simulink model "FirstPass"  (R2017b)
settings: Solver=FixedStepAuto  StartTime=0.0  StopTime=10.0  FixedStep=0.08  RelTol=1e-3
model workspace (MAT data in the model file):
  ContractValidatorBlocksMap = containers.Map
  ContractValidatorBlocksMap.serialization.keys = {'FirstPass/Req_s3_1_2_2_p19_2/validator', 'FirstPass/Req_s3_1_2_2_p19_3/validator', 'FirstPass/contract/validator', 'FirstPass/contract1/validator'}
  ContractValidatorBlocksMap.serialization.values{1}.block = 'FirstPass/Req_s3_1_2_2_p19_2/validator'
  ContractValidatorBlocksMap.serialization.values{1}.assumePorts = 0
  ContractValidatorBlocksMap.serialization.values{1}.guaranteePorts = 1
  ContractValidatorBlocksMap.serialization.values{1}.modeBlocksPorts = 0
  ContractValidatorBlocksMap.serialization.values{1}.portHandles.Inport = 2748.11108398
  ContractValidatorBlocksMap.serialization.values{1}.portHandles.Outport = 2749.11108398
  ContractValidatorBlocksMap.serialization.values{1}.portHandles.Enable = []
  ContractValidatorBlocksMap.serialization.values{1}.portHandles.Trigger = []
  ContractValidatorBlocksMap.serialization.values{1}.portHandles.State = []
  ContractValidatorBlocksMap.serialization.values{1}.portHandles.LConn = []
  ContractValidatorBlocksMap.serialization.values{1}.portHandles.RConn = []
  ContractValidatorBlocksMap.serialization.values{1}.portHandles.Ifaction = []
  ContractValidatorBlocksMap.serialization.values{1}.portHandles.Reset = []
  ContractValidatorBlocksMap.serialization.values{1}.portConnectivity(1).Type = '1'
  ContractValidatorBlocksMap.serialization.values{1}.portConnectivity(1).Position = [365 90]
  ContractValidatorBlocksMap.serialization.values{1}.portConnectivity(1).SrcBlock = 2685.11108398
  ContractValidatorBlocksMap.serialization.values{1}.portConnectivity(1).SrcPort = 0
  ContractValidatorBlocksMap.serialization.values{1}.portConnectivity(1).DstBlock = []
  ContractValidatorBlocksMap.serialization.values{1}.portConnectivity(1).DstPort = []
  ContractValidatorBlocksMap.serialization.values{1}.portConnectivity(2).Type = '1'
  ContractValidatorBlocksMap.serialization.values{1}.portConnectivity(2).Position = [500 90]
  ContractValidatorBlocksMap.serialization.values{1}.portConnectivity(2).SrcBlock = []
  ContractValidatorBlocksMap.serialization.values{1}.portConnectivity(2).SrcPort = []
  ContractValidatorBlocksMap.serialization.values{1}.portConnectivity(2).DstBlock = 2694.11108398
  ContractValidatorBlocksMap.serialization.values{1}.portConnectivity(2).DstPort = 0
  ContractValidatorBlocksMap.serialization.values{2}.block = 'FirstPass/Req_s3_1_2_2_p19_3/validator'
  ContractValidatorBlocksMap.serialization.values{2}.assumePorts = 0
  ContractValidatorBlocksMap.serialization.values{2}.guaranteePorts = 1
  ContractValidatorBlocksMap.serialization.values{2}.modeBlocksPorts = 0
  ContractValidatorBlocksMap.serialization.values{2}.portHandles.Inport = 2746.11132812
  ContractValidatorBlocksMap.serialization.values{2}.portHandles.Outport = 2747.11108398
  ContractValidatorBlocksMap.serialization.values{2}.portHandles.Enable = []
  ContractValidatorBlocksMap.serialization.values{2}.portHandles.Trigger = []
  ContractValidatorBlocksMap.serialization.values{2}.portHandles.State = []
  ContractValidatorBlocksMap.serialization.values{2}.portHandles.LConn = []
  ContractValidatorBlocksMap.serialization.values{2}.portHandles.RConn = []
  ContractValidatorBlocksMap.serialization.values{2}.portHandles.Ifaction = []
  ContractValidatorBlocksMap.serialization.values{2}.portHandles.Reset = []
  ContractValidatorBlocksMap.serialization.values{2}.portConnectivity(1).Type = '1'
  ContractValidatorBlocksMap.serialization.values{2}.portConnectivity(1).Position = [365 75]
  ContractValidatorBlocksMap.serialization.values{2}.portConnectivity(1).SrcBlock = 2703.11108398
  ContractValidatorBlocksMap.serialization.values{2}.portConnectivity(1).SrcPort = 0
  ContractValidatorBlocksMap.serialization.values{2}.portConnectivity(1).DstBlock = []
  ContractValidatorBlocksMap.serialization.values{2}.portConnectivity(1).DstPort = []
  ContractValidatorBlocksMap.serialization.values{2}.portConnectivity(2).Type = '1'
  ContractValidatorBlocksMap.serialization.values{2}.portConnectivity(2).Position = [500 75]
  ContractValidatorBlocksMap.serialization.values{2}.portConnectivity(2).SrcBlock = []
  ContractValidatorBlocksMap.serialization.values{2}.portConnectivity(2).SrcPort = []
  ContractValidatorBlocksMap.serialization.values{2}.portConnectivity(2).DstBlock = 2720.11108398
  ContractValidatorBlocksMap.serialization.values{2}.portConnectivity(2).DstPort = 0
  ContractValidatorBlocksMap.serialization.values{3}.block = 'FirstPass/contract/validator'
  ContractValidatorBlocksMap.serialization.values{3}.assumePorts = 0
  ContractValidatorBlocksMap.serialization.values{3}.guaranteePorts = 1
  ContractValidatorBlocksMap.serialization.values{3}.modeBlocksPorts = 0
  ContractValidatorBlocksMap.serialization.values{3}.portHandles.Inport = 1491.35229492
  ContractValidatorBlocksMap.serialization.values{3}.portHandles.Outport = 1492.35205078
  ContractValidatorBlocksMap.serialization.values{3}.portHandles.Enable = []
  ContractValidatorBlocksMap.serialization.values{3}.portHandles.Trigger = []
  ContractValidatorBlocksMap.serialization.values{3}.portHandles.State = []
  ContractValidatorBlocksMap.serialization.values{3}.portHandles.LConn = []
  ContractValidatorBlocksMap.serialization.values{3}.portHandles.RConn = []
  ContractValidatorBlocksMap.serialization.values{3}.portHandles.Ifaction = []
  ContractValidatorBlocksMap.serialization.values{3}.portHandles.Reset = []
  ContractValidatorBlocksMap.serialization.values{3}.portConnectivity(1).Type = '1'
  ContractValidatorBlocksMap.serialization.values{3}.portConnectivity(1).Position = [365 75]
  ContractValidatorBlocksMap.serialization.values{3}.portConnectivity(1).SrcBlock = 1448.35205078
  ContractValidatorBlocksMap.serialization.values{3}.portConnectivity(1).SrcPort = 0
  ContractValidatorBlocksMap.serialization.values{3}.portConnectivity(1).DstBlock = []
  ContractValidatorBlocksMap.serialization.values{3}.portConnectivity(1).DstPort = []
  ContractValidatorBlocksMap.serialization.values{3}.portConnectivity(2).Type = '1'
  ContractValidatorBlocksMap.serialization.values{3}.portConnectivity(2).Position = [500 75]
  ContractValidatorBlocksMap.serialization.values{3}.portConnectivity(2).SrcBlock = []
  ContractValidatorBlocksMap.serialization.values{3}.portConnectivity(2).SrcPort = []
  ContractValidatorBlocksMap.serialization.values{3}.portConnectivity(2).DstBlock = 1465.35205078
  ContractValidatorBlocksMap.serialization.values{3}.portConnectivity(2).DstPort = 0
  ContractValidatorBlocksMap.serialization.values{4}.block = 'FirstPass/contract1/validator'
  ContractValidatorBlocksMap.serialization.values{4}.assumePorts = 0
  ContractValidatorBlocksMap.serialization.values{4}.guaranteePorts = 1
  ContractValidatorBlocksMap.serialization.values{4}.modeBlocksPorts = 0
  ContractValidatorBlocksMap.serialization.values{4}.portHandles.Inport = 5485.11975098
  ContractValidatorBlocksMap.serialization.values{4}.portHandles.Outport = 5486.11975098
  ContractValidatorBlocksMap.serialization.values{4}.portHandles.Enable = []
  ContractValidatorBlocksMap.serialization.values{4}.portHandles.Trigger = []
  ContractValidatorBlocksMap.serialization.values{4}.portHandles.State = []
  ContractValidatorBlocksMap.serialization.values{4}.portHandles.LConn = []
  ContractValidatorBlocksMap.serialization.values{4}.portHandles.RConn = []
  ContractValidatorBlocksMap.serialization.values{4}.portHandles.Ifaction = []
  ContractValidatorBlocksMap.serialization.values{4}.portHandles.Reset = []
  ContractValidatorBlocksMap.serialization.values{4}.portConnectivity(1).Type = '1'
  ContractValidatorBlocksMap.serialization.values{4}.portConnectivity(1).Position = [365 75]
  ContractValidatorBlocksMap.serialization.values{4}.portConnectivity(1).SrcBlock = 5292.11987305
  ContractValidatorBlocksMap.serialization.values{4}.portConnectivity(1).SrcPort = 0
  ContractValidatorBlocksMap.serialization.values{4}.portConnectivity(1).DstBlock = []
  ContractValidatorBlocksMap.serialization.values{4}.portConnectivity(1).DstPort = []
  ContractValidatorBlocksMap.serialization.values{4}.portConnectivity(2).Type = '1'
  ContractValidatorBlocksMap.serialization.values{4}.portConnectivity(2).Position = [500 75]
  ContractValidatorBlocksMap.serialization.values{4}.portConnectivity(2).SrcBlock = []
  ContractValidatorBlocksMap.serialization.values{4}.portConnectivity(2).SrcPort = []
  ContractValidatorBlocksMap.serialization.values{4}.portConnectivity(2).DstBlock = 5462.12011719
  ContractValidatorBlocksMap.serialization.values{4}.portConnectivity(2).DstPort = 0
  ContractValidatorBlocksMap.serialization.uniformity = 0
  ContractValidatorBlocksMap.serialization.keyType = 'char'
  ContractValidatorBlocksMap.serialization.valueType = 'any'
undefined symbols (not defined in the file or in its folder): contractAfterSimulation, contractBeforeSimulation, ContractBlock, ContractGuaranteeBlock, ContractValidatorBlock, Req_s3_1_2_2_p19_2, saveValidatorParameters
libraries: sldvlib x2
settings Model: Creator=hbourbou  LastModifiedBy=hbourbou

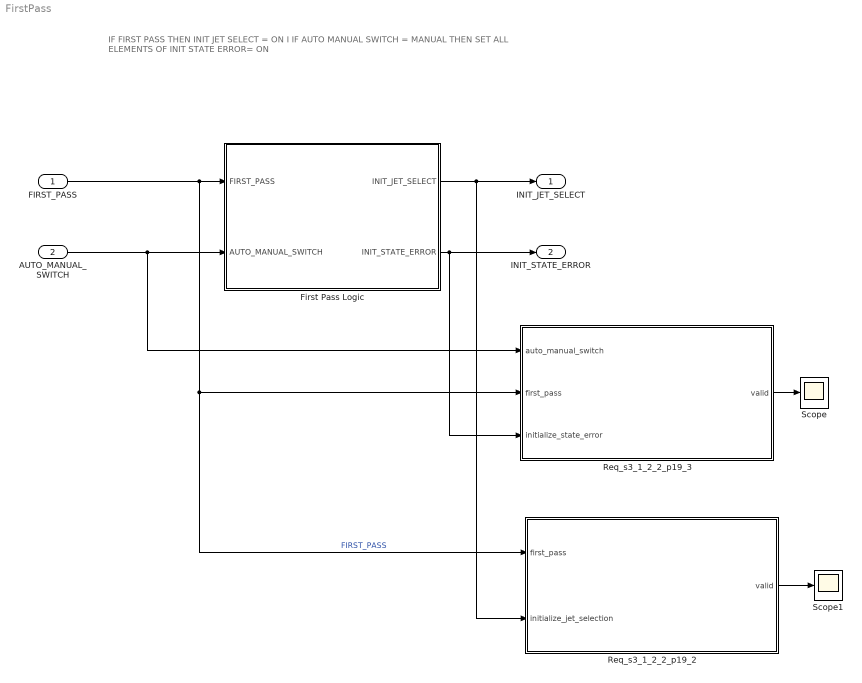
== system FirstPass ==
  note: IF FIRST PASS THEN
      | INIT JET SELECT = ON I
      | IF AUTO MANUAL SWITCH = MANUAL THEN
      | SET ALL ELEMENTS OF INIT STATE ERROR= ON
  FIRST_PASS : Inport  OutDataTypeStr=boolean
  AUTO_MANUAL_SWITCH : Inport  Port=2  OutDataTypeStr=boolean  PortDimensions=1
  First Pass Logic : Subsystem
  Req_s3_1_2_2_p19_2 : Subsystem  mask(ContractBlock){ContractBlockType=Req_s3_1_2_2_p19_2}
      mask init:
      | set_param(gcb, 'LinkStatus', 'none');
      settings: CopyFcn=set_param(gcb, 'LinkStatus', 'none');
      mask DialogControl DescTextVar Prompt: Contract block
      mask Display:
      | text(0.5, 0.5, '{\bf\fontsize{20}Contract}', 'hor', 'center', 'texmode','on');
      | blocks = find_system(gcb, 'LookUnderMasks','all', 'SearchDepth',1,'BlockType','Inport');
      | for i = 1 : length(blocks)
      |     blockName = get_param(blocks(i), 'Name');
      |     [path, blockName] = fileparts(char(blockName));
      |     port_label('input', i, blockName);
      | end
      | 
      | blocks = find_system(gcb, 'LookUnderMasks','all', 'SearchDepth',1,'BlockType','Outport');
      | for i = 1 : length(blocks)
      |     blockName = get_param(blocks(i), 'Name');
      |     [path, blockName] = fileparts(char(blockName));
      |     port_label('output', i, blockName);
      | end
  Req_s3_1_2_2_p19_3 : Subsystem  mask(ContractBlock){ContractBlockType=ContractBlock}
      mask init:
      | set_param(gcb, 'LinkStatus', 'none');
      settings: CopyFcn=set_param(gcb, 'LinkStatus', 'none');
      mask DialogControl DescTextVar Prompt: Contract block
      mask Display:
      | text(0.5, 0.5, '{\bf\fontsize{20}Contract}', 'hor', 'center', 'texmode','on');
      | blocks = find_system(gcb, 'LookUnderMasks','all', 'SearchDepth',1,'BlockType','Inport');
      | for i = 1 : length(blocks)
      |     blockName = get_param(blocks(i), 'Name');
      |     [path, blockName] = fileparts(char(blockName));
      |     port_label('input', i, blockName);
      | end
      | 
      | blocks = find_system(gcb, 'LookUnderMasks','all', 'SearchDepth',1,'BlockType','Outport');
      | for i = 1 : length(blocks)
      |     blockName = get_param(blocks(i), 'Name');
      |     [path, blockName] = fileparts(char(blockName));
      |     port_label('output', i, blockName);
      | end
  Scope : Scope
  Scope1 : Scope
  INIT_JET_SELECT : Outport
  INIT_STATE_ERROR : Outport  Port=2
  wires:
  FIRST_PASS/1 -> Req_s3_1_2_2_p19_2/1(first_pass), Req_s3_1_2_2_p19_3/2(first_pass), First Pass Logic/1(FIRST_PASS)  "FIRST_PASS"
  AUTO_MANUAL_SWITCH/1 -> Req_s3_1_2_2_p19_3/1(auto_manual_switch), First Pass Logic/2(AUTO_MANUAL_SWITCH)
  First Pass Logic/1(INIT_JET_SELECT) -> Req_s3_1_2_2_p19_2/2(initialize_jet_selection), INIT_JET_SELECT/1
  First Pass Logic/2(INIT_STATE_ERROR) -> Req_s3_1_2_2_p19_3/3(initialize_state_error), INIT_STATE_ERROR/1
  Req_s3_1_2_2_p19_3/1(valid) -> Scope/1
  Req_s3_1_2_2_p19_2/1(valid) -> Scope1/1

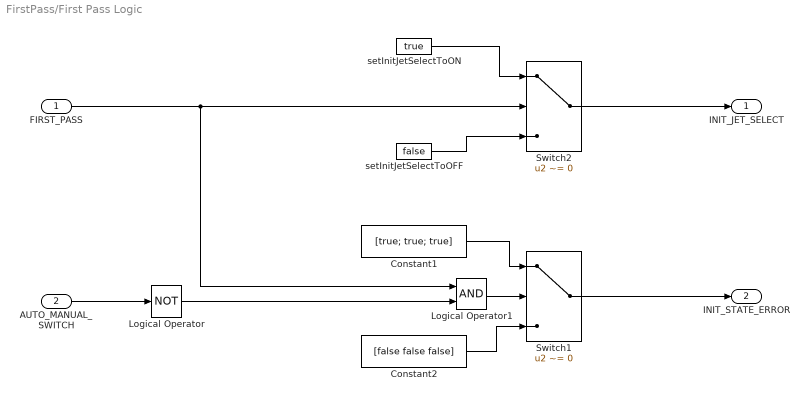
== system FirstPass/First Pass Logic ==
  FIRST_PASS : Inport
  AUTO_MANUAL_SWITCH : Inport  Port=2
  Constant1 : Constant  Value=[true; true; true]  OutDataTypeStr=boolean
  Constant2 : Constant  Value=[false false false]  OutDataTypeStr=boolean
  Logical Operator : Logic  Operator=NOT  AllPortsSameDT=off  OutDataTypeStr=boolean
  Logical Operator1 : Logic  AllPortsSameDT=off  OutDataTypeStr=boolean
  Switch1 : Switch  Criteria=u2 ~= 0
  Switch2 : Switch  Criteria=u2 ~= 0
  setInitJetSelectToOFF : Constant  Value=false  OutDataTypeStr=boolean
  setInitJetSelectToON : Constant  Value=true  OutDataTypeStr=boolean
  INIT_JET_SELECT : Outport
  INIT_STATE_ERROR : Outport  Port=2
  wires:
  Constant1/1 -> Switch1/1
  Switch1/1 -> INIT_STATE_ERROR/1
  Constant2/1 -> Switch1/3
  Switch2/1 -> INIT_JET_SELECT/1
  setInitJetSelectToON/1 -> Switch2/1
  setInitJetSelectToOFF/1 -> Switch2/3
  Logical Operator1/1 -> Switch1/2
  AUTO_MANUAL_SWITCH/1 -> Logical Operator/1
  Logical Operator/1 -> Logical Operator1/2
  FIRST_PASS/1 -> Logical Operator1/1, Switch2/2

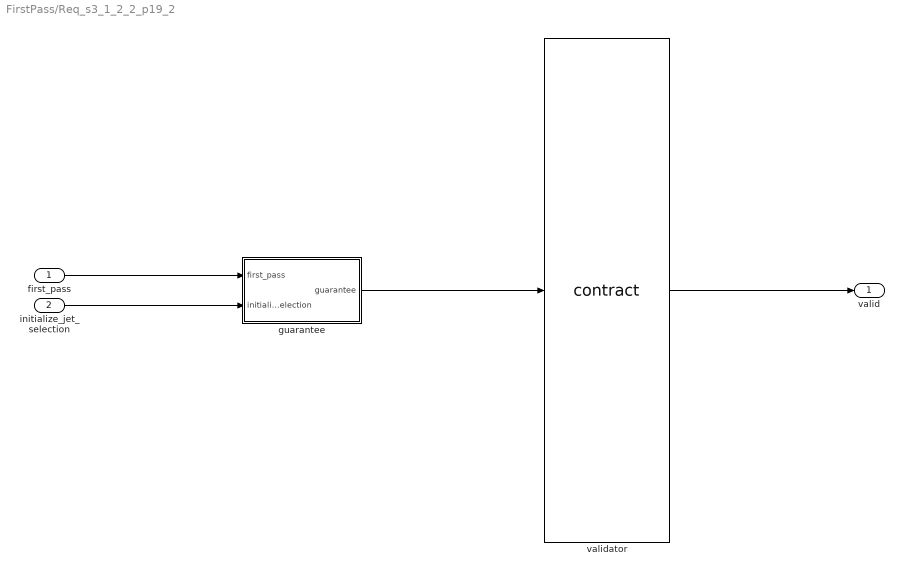
== system FirstPass/Req_s3_1_2_2_p19_2 ==
  first_pass : Inport
  initialize_jet_selection : Inport  Port=2
  guarantee : Subsystem  mask(ContractGuaranteeBlock){ContractBlockType=ContractGuaranteeBlock}
      mask init:
      | set_param(gcb, 'LinkStatus', 'none');
      mask DialogControl DescTextVar Prompt: Guarantee block
  validator : M-S-Function  LoadFcn=saveValidatorParameters(gcb);  InitFcn=contractBeforeSimulation();  StopFcn=contractAfterSimulation();  FunctionName=contract  mask(ContractValidatorBlock){assumePorts=0, guaranteePorts=1, modePorts=0, ContractBlockType=ContractValidatorBlock, createInportsCheckbox=off}
      mask prompts: assumePorts "Assume ports     :"; guaranteePorts "Guarantee ports :"; modePorts "Mode ports        :"; createInportsCheckbox "Create inports and connect them automatically"
      mask init:
      | set_param(gcb,'LinkStatus','none');
      | contract_callback('inputs_callback',gcb);
      mask DialogControl DescTextVar Prompt: The validator block implements the following logic: <br> <br> <b>Sofar</b>(assume<sub>1</sub> <b>&#8743;</b> assume<sub>2</sub> <b>&#8743;</b> ... assume<sub>k</sub>) <b>&rarr;</b> (guarantee<sub>1</sub> <b>&#8743;</b> guarantee<sub>2</sub> <b>&#8743;</b> ... guarantee<sub>m</sub> <b>&#8743;</b>  mode<sub>1</sub> <b>&#8743;</b> mode<sub>2</sub> <b>&#8743;</b> ... <b>&#8743;</b> mode<sub>n</sub> )<br> where mode<sub>i</sub> = require<sub>i</sub> <b>&rarr;</b> ensure<sub>i</sub>
      mask Display:
      | color('black');
      | port_label('input',1,'guarantee');
      | port_label('output',1,'valid');
  valid : Outport
  wires:
  initialize_jet_selection/1 -> guarantee/2(initialize_jet_selection)
  first_pass/1 -> guarantee/1(first_pass)
  validator/1 -> valid/1
  guarantee/1(guarantee) -> validator/1

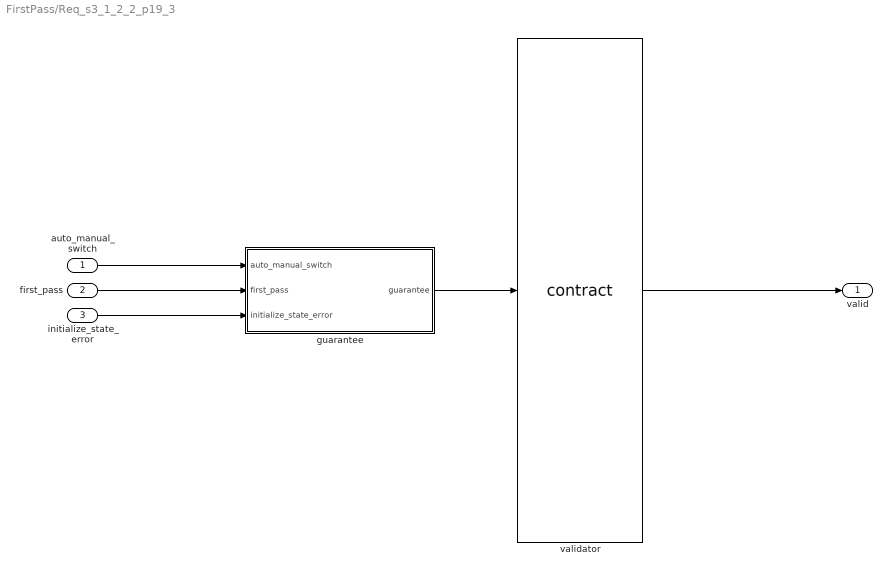
== system FirstPass/Req_s3_1_2_2_p19_3 ==
  auto_manual_switch : Inport
  first_pass : Inport  Port=2
  initialize_state_error : Inport  Port=3
  guarantee : Subsystem  mask(ContractGuaranteeBlock){ContractBlockType=ContractGuaranteeBlock}
      mask init:
      | set_param(gcb, 'LinkStatus', 'none');
      mask DialogControl DescTextVar Prompt: Guarantee block
  validator : M-S-Function  LoadFcn=saveValidatorParameters(gcb);  InitFcn=contractBeforeSimulation();  StopFcn=contractAfterSimulation();  FunctionName=contract  mask(ContractValidatorBlock){assumePorts=0, guaranteePorts=1, modePorts=0, ContractBlockType=ContractValidatorBlock, createInportsCheckbox=on}
      mask prompts: assumePorts "Assume ports     :"; guaranteePorts "Guarantee ports :"; modePorts "Mode ports        :"; createInportsCheckbox "Create inports and connect them automatically"
      mask init:
      | set_param(gcb,'LinkStatus','none');
      | contract_callback('inputs_callback',gcb);
      mask DialogControl DescTextVar Prompt: The validator block implements the following logic: <br> <br> <b>Sofar</b>(assume<sub>1</sub> <b>&#8743;</b> assume<sub>2</sub> <b>&#8743;</b> ... assume<sub>k</sub>) <b>&rarr;</b> (guarantee<sub>1</sub> <b>&#8743;</b> guarantee<sub>2</sub> <b>&#8743;</b> ... guarantee<sub>m</sub> <b>&#8743;</b>  mode<sub>1</sub> <b>&#8743;</b> mode<sub>2</sub> <b>&#8743;</b> ... <b>&#8743;</b> mode<sub>n</sub> )<br> where mode<sub>i</sub> = require<sub>i</sub> <b>&rarr;</b> ensure<sub>i</sub>
      mask Display:
      | color('black');
      | port_label('input',1,'guarantee');
      | port_label('output',1,'valid');
  valid : Outport
  wires:
  first_pass/1 -> guarantee/2(first_pass)
  auto_manual_switch/1 -> guarantee/1(auto_manual_switch)
  validator/1 -> valid/1
  guarantee/1(guarantee) -> validator/1
  initialize_state_error/1 -> guarantee/3(initialize_state_error)

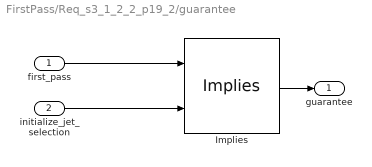
== system FirstPass/Req_s3_1_2_2_p19_2/guarantee ==
  first_pass : Inport
  initialize_jet_selection : Inport  Port=2
  Implies : sldvlib/Verification Utilities/Implies
      settings: SourceProductName=Simulink Design Verifier  SourceProductBaseCode=DV
  guarantee : Outport  OutDataTypeStr=boolean
  wires:
  Implies/1 -> guarantee/1
  first_pass/1 -> Implies/1
  initialize_jet_selection/1 -> Implies/2

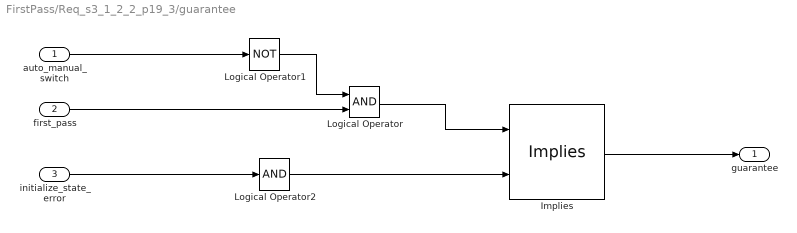
== system FirstPass/Req_s3_1_2_2_p19_3/guarantee ==
  auto_manual_switch : Inport
  first_pass : Inport  Port=2
  initialize_state_error : Inport  Port=3
  Implies : sldvlib/Verification Utilities/Implies
      settings: SourceProductName=Simulink Design Verifier  SourceProductBaseCode=DV
  Logical Operator : Logic  AllPortsSameDT=off  OutDataTypeStr=boolean
  Logical Operator1 : Logic  Operator=NOT  Inputs=1  AllPortsSameDT=off  OutDataTypeStr=boolean
  Logical Operator2 : Logic  Inputs=1  AllPortsSameDT=off  OutDataTypeStr=boolean
  guarantee : Outport  OutDataTypeStr=boolean
  wires:
  Implies/1 -> guarantee/1
  initialize_state_error/1 -> Logical Operator2/1
  Logical Operator/1 -> Implies/1
  first_pass/1 -> Logical Operator/2
  Logical Operator1/1 -> Logical Operator/1
  auto_manual_switch/1 -> Logical Operator1/1
  Logical Operator2/1 -> Implies/2
